simulink model "MBD_W1_P7"  (R2020a)
settings: Solver=VariableStepAuto  StartTime=0.0  StopTime=10.0  RelTol=1e-3
settings Model: Creator=Atri Mondal  LastModifiedBy=Atri Mondal

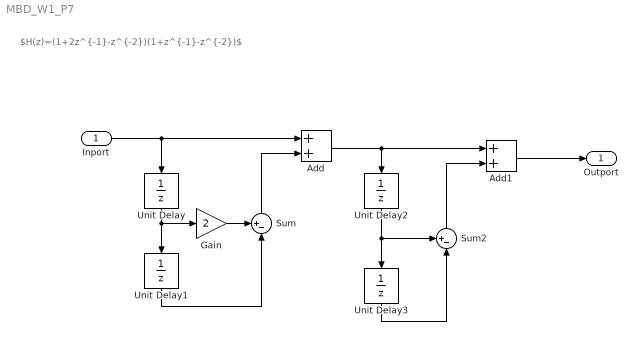
== system MBD_W1_P7 ==
  note: $H(z)=(1+2z^{-1}-z^{-2})(1+z^{-1}-z^{-2})$
  Inport : Inport
  Add : Sum
  Add1 : Sum
  Gain : Gain  Gain=2
  Sum : Sum  Inputs=+-|
  Sum2 : Sum  Inputs=+-|
  Unit Delay{,1..3} (4 alike) : UnitDelay  SampleTime=-1  HasFrameUpgradeWarning=on
  Outport : Outport
  wires:
  Inport/1 -> Unit Delay/1, Add/1
  Unit Delay/1 -> Gain/1, Unit Delay1/1
  Unit Delay1/1 -> Sum/2
  Sum/1 -> Add/2
  Sum2/1 -> Add1/2
  Unit Delay3/1 -> Sum2/2
  Add/1 -> Add1/1, Unit Delay2/1
  Unit Delay2/1 -> Sum2/1, Unit Delay3/1
  Gain/1 -> Sum/1
  Add1/1 -> Outport/1
